simulink library "Driveline_Axle1_Differential"  (R2019a)
settings: Solver=VariableStepAuto  StartTime=0.0  StopTime=10.0  RelTol=1e-3
libraries: sm_car_lib x3, fl_lib x1, sdl_lib x1
Description:
  | Component of Simscape Vehicle Templates Library
  | 
  | Copyright 2018-2020 The MathWorks, Inc.
settings Model: Creator=smiller  LastModifiedBy=smiller
settings DataIOCC: ReturnWorkspaceOutputs=off
settings DebuggingCC: ArithmeticOperatorsInVariantConditions=warning

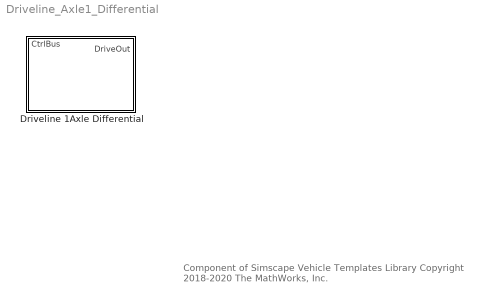
== system Driveline_Axle1_Differential ==
  note: Component of Simscape Vehicle Templates Library
      | Copyright 2018-2020 The MathWorks, Inc.
  Driveline 1Axle Differential : Subsystem  Tag=PublishSubsystem  VariantControl=IndepFRDiffFDiffR  mask(Driveline, Independent Front and Rear){InitTriggerDropdown=0}
      mask prompts: InitTriggerDropdown "Initialization Trigger Dropdown"
      mask help: Models independent drivelines for front and rear axles.
      mask init:
      | curblk = gcb;
      | 
      | % Trigger Mask Initialization for 
      | % variant subsystems below this level
      | sm_car_lib_maskInitTrigger(curblk)
      mask TypeOptions InitTriggerDropdown: 0 | 1

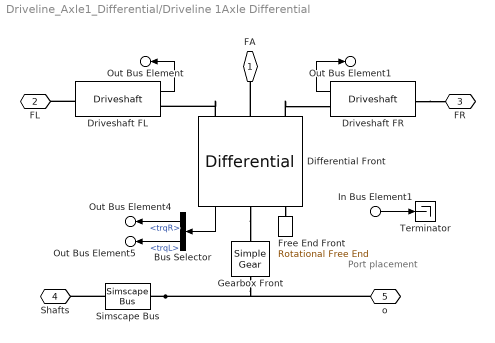
== system Driveline_Axle1_Differential/Driveline 1Axle Differential ==
  note: Port
      | placement
  In Bus Element1 : Inport  PortName=CtrlBus
  Bus Selector : BusSelector  OutputSignals=trqR,trqL
  Differential Front : sm_car_lib/Driveline/Differential  VariantControl=Variant1  Differential=Driveline.DifferentialF  VariantLabel=Driveline.DifferentialF.class.Value  InitTriggerDropdown=0
      settings: AttributesFormatString=%<ActiveVariant>
  Driveshaft FL : sm_car_lib/Driveline/Driveshaft  VariantControl=Variant1  popup_leftRight=Left  Driveshaft=Driveline.DriveshaftFL  VariantLabel=Driveline.DriveshaftFL.class.Value  InitTriggerDropdown=0
      settings: AttributesFormatString=%<ActiveVariant>
  Driveshaft FR : sm_car_lib/Driveline/Driveshaft  VariantControl=Variant1  popup_leftRight=Right  Driveshaft=Driveline.DriveshaftFR  VariantLabel=Driveline.DriveshaftFR.class.Value  InitTriggerDropdown=0
      settings: AttributesFormatString=%<ActiveVariant>
  Free End Front : fl_lib/Mechanical/Rotational Elements/Rotational Free End  w_specify=off  w_priority=None  w=0 rad/s  w_nominal_specify=off  w_nominal_unit=rad/s  w_nominal_value=1
      settings: SourceProductName=Simscape  SourceProductBaseCode=SS
  Gearbox Front : sdl_lib/Gears/Simple Gear  ratio=Driveline.GearboxF.ratio.Value  rotation_direction=1  friction_model=1  T_noload=0.1 N*m  T_nom=5 N*m  efficiency_nom=0.8  efficiency=0.8  mu_visc=[0, 0] N*m/(rad/s)  w_thr=0.01 rad/s  pwr_thr=0.001 W  enable_faults=0  efficiency_fault=0.05  external_fault=simscape.enum.onoff.off  temporal_fault=0  fault_time=5 s  fault_angles=pi / 12 rad  report_fault=1  temperature_TLU=[280, 300, 320] K  load_TLU=[1, 5, 10] N*m  efficiency_TLU=[.95, .9, .85]  efficiency_TLU2=[.85, .8, .75; .95, .9, .85; .85, .8, .7]  thermal_mass=50 J/K  T_init=300 K
      settings: SourceProductName=Simscape Driveline
  Simscape Bus : SimscapeBus  HierarchyStrings=ShaftF
  Terminator : Terminator
  FA : PMIOPort  Side=Left
  FL : PMIOPort  Port=2  Side=Left
  FR : PMIOPort  Port=3  Side=Right
  Shafts : PMIOPort  Port=4  Side=Left
  o : PMIOPort  Port=5  Side=Right
  Out Bus Element4 : Outport  PortName=DriveOut  Element=MDriveshaftFL
  Out Bus Element5 : Outport  PortName=DriveOut  Element=MDriveshaftFR
  Out Bus Element : Outport  PortName=DriveOut  Element=anDriveshaftFL
  Out Bus Element1 : Outport  PortName=DriveOut  Element=anDriveshaftFR
  wires:
  Driveshaft FR/1 -> Out Bus Element1/1
  Driveshaft FL/1 -> Out Bus Element/1
  Differential Front/1 -> Bus Selector/1
  Bus Selector/1 -> Out Bus Element4/1  "<trqR>"
  Bus Selector/2 -> Out Bus Element5/1  "<trqL>"
  In Bus Element1/1 -> Terminator/1
  connections:
  Simscape Bus/LConn1 -- Gearbox Front/LConn1 -- o/RConn1
  Differential Front/RConn2 -- Free End Front/LConn1
  Differential Front/LConn1 -- Driveshaft FL/RConn1
  Differential Front/LConn3 -- Driveshaft FR/RConn1
  Driveshaft FR/LConn1 -- FR/RConn1
  Driveshaft FL/LConn1 -- FL/RConn1
  Differential Front/LConn2 -- FA/RConn1
  Differential Front/RConn1 -- Gearbox Front/RConn1
  Simscape Bus/RConn1 -- Shafts/RConn1
